simulink model "PTMotorCU"  (Simulink 8.7)
settings: Solver=ode45  StartTime=0.0  StopTime=inf  RelTol=1e-3
PreLoadFcn:
  | xData = [0 13.5 21 35 50 100];
  | yData = [150 150 95 57 39 20];
InitFcn:
  | xData = [0 0.128];
  | yData = [150 150];
libraries: simulink x6
(part 2 of 2)

== system PTMotorCU/CarMaker/IPG Vehicle/CarAndTrailer/Forces/Tires ==
  note: The TireXX_Out signals will only be used if FileIdent is "CarMaker-Tire-CM4SL" in the tire parameter file!
      | An example parameter file can be found in Data/Tire/DT_CM4SL_UserTire.
  Sync_In : Inport
  TireFL_In : Inport  Port=2
  TireFR_In : Inport  Port=3
  TireRL_In : Inport  Port=4
  TireRR_In : Inport  Port=5
  Bus Creator{1..4} (4 alike) : BusCreator  Inputs=11
  Demux{1..3,8} (4 alike) : Demux  Outputs=7
  TireFL : Subsystem
  TireFR : Subsystem
  TireRL : Subsystem
  TireRR : Subsystem
  TireFL_Out : Outport
  TireFR_Out : Outport  Port=2
  TireRL_Out : Outport  Port=3
  TireRR_Out : Outport  Port=4
  wires:
  Sync_In/1 -> TireRR/1(Sync_In), TireRL/1(Sync_In), TireFR/1(Sync_In), TireFL/1(Sync_In)
  Bus Creator4/1 -> TireRR_Out/1
  Bus Creator2/1 -> TireRL_Out/1
  Bus Creator1/1 -> TireFR_Out/1
  Demux3/5 -> TireRR/6(Rim_turnv)  "Tire_In Rim_turnv"
  Demux3/4 -> TireRR/5(Rim_rotv)  "Tire_In Rim_rotv"
  Demux3/1 -> TireRR/2(Load)  "Tire_In Load"
  Demux3/7 -> TireRR/8(muRoad)  "Tire_In mu"
  Demux3/6 -> TireRR/7(InclinAngle)  "Tire_In Camber"
  Demux3/2 -> TireRR/3(vxtrans)  "Tire_In vxtrans"
  Demux3/3 -> TireRR/4(vytrans)  "Tire_In vytrans"
  TireRR/11(AlignTrq) -> Bus Creator4/11  "Tire_Out AlignTrq"
  TireRR/10(RollResist) -> Bus Creator4/10  "Tire_Out RollResist"
  TireRR/9(OverturnTrq) -> Bus Creator4/9  "Tire_Out OverturnTrq"
  TireRR/8(LoadFrc) -> Bus Creator4/8  "Tire_Out LoadFrc"
  TireRR/7(SideFrc) -> Bus Creator4/7  "Tire_Out SideFrc"
  TireRR/6(LongFrc) -> Bus Creator4/6  "Tire_Out LongFrc"
  TireRR/5(vBelt) -> Bus Creator4/5  "Tire_Out vBelt"
  TireRR/4(rBelt_eff) -> Bus Creator4/4  "Tire_Out rBelt_eff"
  TireRR/3(TurnSlp) -> Bus Creator4/3  "Tire_Out TurnSlp"
  TireRR/1(Slp) -> Bus Creator4/1  "Tire_Out Slp"
  TireRR/2(Alpha) -> Bus Creator4/2  "Tire_Out Alpha"
  Demux2/5 -> TireRL/6(Rim_turnv)  "Tire_In Rim_turnv"
  Demux2/4 -> TireRL/5(Rim_rotv)  "Tire_In Rim_rotv"
  Demux2/1 -> TireRL/2(Load)  "Tire_In Load"
  Demux2/7 -> TireRL/8(muRoad)  "Tire_In mu"
  Demux2/6 -> TireRL/7(InclinAngle)  "Tire_In Camber"
  Demux2/2 -> TireRL/3(vxtrans)  "Tire_In vxtrans"
  Demux2/3 -> TireRL/4(vytrans)  "Tire_In vytrans"
  TireRL/11(AlignTrq) -> Bus Creator2/11  "Tire_Out AlignTrq"
  TireRL/10(RollResist) -> Bus Creator2/10  "Tire_Out RollResist"
  TireRL/9(OverturnTrq) -> Bus Creator2/9  "Tire_Out OverturnTrq"
  TireRL/8(LoadFrc) -> Bus Creator2/8  "Tire_Out LoadFrc"
  TireRL/7(SideFrc) -> Bus Creator2/7  "Tire_Out SideFrc"
  TireRL/6(LongFrc) -> Bus Creator2/6  "Tire_Out LongFrc"
  TireRL/5(vBelt) -> Bus Creator2/5  "Tire_Out vBelt"
  TireRL/4(rBelt_eff) -> Bus Creator2/4  "Tire_Out rBelt_eff"
  TireRL/3(TurnSlp) -> Bus Creator2/3  "Tire_Out TurnSlp"
  TireRL/1(Slp) -> Bus Creator2/1  "Tire_Out Slp"
  TireRL/2(Alpha) -> Bus Creator2/2  "Tire_Out Alpha"
  Demux1/5 -> TireFR/6(Rim_turnv)  "Tire_In Rim_turnv"
  Demux1/4 -> TireFR/5(Rim_rotv)  "Tire_In Rim_rotv"
  Demux1/1 -> TireFR/2(Load)  "Tire_In Load"
  Demux1/7 -> TireFR/8(muRoad)  "Tire_In mu"
  Demux1/6 -> TireFR/7(InclinAngle)  "Tire_In Camber"
  Demux1/2 -> TireFR/3(vxtrans)  "Tire_In vxtrans"
  Demux1/3 -> TireFR/4(vytrans)  "Tire_In vytrans"
  TireFR/11(AlignTrq) -> Bus Creator1/11  "Tire_Out AlignTrq"
  TireFR/10(RollResist) -> Bus Creator1/10  "Tire_Out RollResist"
  TireFR/9(OverturnTrq) -> Bus Creator1/9  "Tire_Out OverturnTrq"
  TireFR/8(LoadFrc) -> Bus Creator1/8  "Tire_Out LoadFrc"
  TireFR/7(SideFrc) -> Bus Creator1/7  "Tire_Out SideFrc"
  TireFR/6(LongFrc) -> Bus Creator1/6  "Tire_Out LongFrc"
  TireFR/5(vBelt) -> Bus Creator1/5  "Tire_Out vBelt"
  TireFR/4(rBelt_eff) -> Bus Creator1/4  "Tire_Out rBelt_eff"
  TireFR/3(TurnSlp) -> Bus Creator1/3  "Tire_Out TurnSlp"
  TireFR/1(Slp) -> Bus Creator1/1  "Tire_Out Slp"
  TireFR/2(Alpha) -> Bus Creator1/2  "Tire_Out Alpha"
  Demux8/5 -> TireFL/6(Rim_turnv)  "Tire_In Rim_turnv"
  Demux8/4 -> TireFL/5(Rim_rotv)  "Tire_In Rim_rotv"
  TireFL_In/1 -> Demux8/1
  Demux8/1 -> TireFL/2(Load)  "Tire_In Load"
  Demux8/7 -> TireFL/8(muRoad)  "Tire_In mu"
  Demux8/6 -> TireFL/7(InclinAngle)  "Tire_In Camber"
  Demux8/2 -> TireFL/3(vxtrans)  "Tire_In vxtrans"
  Demux8/3 -> TireFL/4(vytrans)  "Tire_In vytrans"
  TireFL/11(AlignTrq) -> Bus Creator3/11  "Tire_Out AlignTrq"
  TireFL/10(RollResist) -> Bus Creator3/10  "Tire_Out RollResist"
  TireFL/9(OverturnTrq) -> Bus Creator3/9  "Tire_Out OverturnTrq"
  TireFL/8(LoadFrc) -> Bus Creator3/8  "Tire_Out LoadFrc"
  TireFL/7(SideFrc) -> Bus Creator3/7  "Tire_Out SideFrc"
  TireFL/6(LongFrc) -> Bus Creator3/6  "Tire_Out LongFrc"
  TireFL/5(vBelt) -> Bus Creator3/5  "Tire_Out vBelt"
  TireFL/4(rBelt_eff) -> Bus Creator3/4  "Tire_Out rBelt_eff"
  TireFL/3(TurnSlp) -> Bus Creator3/3  "Tire_Out TurnSlp"
  TireFL/1(Slp) -> Bus Creator3/1  "Tire_Out Slp"
  TireFL/2(Alpha) -> Bus Creator3/2  "Tire_Out Alpha"
  Bus Creator3/1 -> TireFL_Out/1
  TireFR_In/1 -> Demux1/1
  TireRL_In/1 -> Demux2/1
  TireRR_In/1 -> Demux3/1

== system PTMotorCU/CarMaker/IPG Vehicle/CarAndTrailer/Forces/Vehicle Forces ==
  Sync_In : Inport
  Bus Creator1 : BusCreator  Inputs=12
  Bus Creator8 : BusCreator  Inputs=16
  BusCreator1 : BusCreator  Inputs=4
  BusCreator2 : BusCreator  Inputs=9
  Demux : Demux  Outputs=16
  Demux1 : Demux  Outputs=12
  Demux2 : Demux  Outputs=13
  Forces : S-Function  FunctionName=CM_Sfun  Parameters='Forces'  SFunctionDeploymentMode=off  EnableBusSupport=off
  Terminator : Terminator
  Sync_Out : Outport
  Car.Virtual : Outport  Port=2
  Car.Aero : Outport  Port=3
  Car.Load : Outport  Port=4
  wires:
  BusCreator1/1 -> Terminator/1  "Aero IF (in)"
  Demux2/13 -> BusCreator2/9  "car Aero Trq_1 z"
  Demux2/12 -> BusCreator2/8  "car Aero Trq_1 y"
  Demux2/11 -> BusCreator2/7  "car Aero Trq_1 x"
  Demux2/10 -> BusCreator2/6  "car Aero Frc_1 z"
  Demux2/9 -> BusCreator2/5  "car Aero Frc_1 y"
  Demux2/8 -> BusCreator2/4  "car Aero Frc_1 x"
  Demux2/7 -> BusCreator2/3  "car Aero PoA_1 z"
  Demux2/6 -> BusCreator2/2  "car Aero PoA_1 y"
  Demux2/5 -> BusCreator2/1  "car Aero PoA_1 x"
  Demux2/4 -> BusCreator1/4  "car Aero tau_1"
  Demux2/3 -> BusCreator1/3  "car Aero ApproachVel_1 z"
  Demux2/2 -> BusCreator1/2  "car Aero ApproachVel_1 y"
  Demux2/1 -> BusCreator1/1  "car Aero ApproachVel_1 x"
  Demux/16 -> Bus Creator8/16  "Car Load_3 tz"
  Demux/15 -> Bus Creator8/15  "Car Load_3 ty"
  Demux/14 -> Bus Creator8/14  "Car Load_3 tx"
  Demux/13 -> Bus Creator8/13  "Car Load_3 mass"
  Demux1/12 -> Bus Creator1/12  "Car Virtual Trq_0 z"
  Demux1/11 -> Bus Creator1/11  "Car Virtual Trq_0 y"
  Demux1/10 -> Bus Creator1/10  "Car Virtual Trq_0 x"
  Demux1/9 -> Bus Creator1/9  "Car Virtual Trq_1 z"
  Demux1/8 -> Bus Creator1/8  "Car Virtual Trq_1 y"
  Demux1/7 -> Bus Creator1/7  "Car Virtual Trq_1 x"
  Demux1/6 -> Bus Creator1/6  "Car Virtual Frc_0 z"
  Demux1/5 -> Bus Creator1/5  "Car Virtual Frc_0 y"
  Demux1/4 -> Bus Creator1/4  "Car Virtual Frc_0 x"
  Sync_In/1 -> Forces/1
  Forces/1 -> Sync_Out/1
  BusCreator2/1 -> Car.Aero/1
  Demux1/1 -> Bus Creator1/1  "Car Virtual Frc_1 x"
  Demux1/2 -> Bus Creator1/2  "Car Virtual Frc_1 y"
  Demux1/3 -> Bus Creator1/3  "Car Virtual Frc_1 z"
  Forces/3 -> Demux2/1
  Forces/2 -> Demux1/1
  Bus Creator1/1 -> Car.Virtual/1
  Bus Creator8/1 -> Car.Load/1
  Demux/1 -> Bus Creator8/1  "Car Load_0 mass"
  Demux/2 -> Bus Creator8/2  "Car Load_0 tx"
  Demux/3 -> Bus Creator8/3  "Car Load_0 ty"
  Demux/4 -> Bus Creator8/4  "Car Load_0 tz"
  Demux/5 -> Bus Creator8/5  "Car Load_1 mass"
  Demux/6 -> Bus Creator8/6  "Car Load_1 tx"
  Demux/7 -> Bus Creator8/7  "Car Load_1 ty"
  Demux/8 -> Bus Creator8/8  "Car Load_1 tz"
  Demux/9 -> Bus Creator8/9  "Car Load_2 mass"
  Demux/10 -> Bus Creator8/10  "Car Load_2 tx"
  Demux/11 -> Bus Creator8/11  "Car Load_2 ty"
  Demux/12 -> Bus Creator8/12  "Car Load_2 tz"
  Forces/4 -> Demux/1

== system PTMotorCU/CarMaker/IPG Vehicle/CarAndTrailer/Trailer/CreateBus Car.Hitch.FrcTrq ==
  In1 : Inport
  Bus Creator7 : BusCreator  Inputs=6
  Demux7 : Demux  Outputs=6
  Out1 : Outport
  wires:
  In1/1 -> Demux7/1
  Bus Creator7/1 -> Out1/1
  Demux7/6 -> Bus Creator7/6  "Car Hitch Trq2Car z"
  Demux7/5 -> Bus Creator7/5  "Car Hitch Trq2Car y"
  Demux7/4 -> Bus Creator7/4  "Car Hitch Trq2Car x"
  Demux7/3 -> Bus Creator7/3  "Car Hitch Frc2Car z"
  Demux7/2 -> Bus Creator7/2  "Car Hitch Frc2Car y"
  Demux7/1 -> Bus Creator7/1  "Car Hitch Frc2Car x"

== system PTMotorCU/CarMaker/IPG Vehicle/CarAndTrailer/Trailer/CreateBus Vhcl.Motion ==
  In1 : Inport
  BusCreator : BusCreator  Inputs=15
  Demux : Demux  Outputs=15
  Out1 : Outport
  wires:
  Demux/15 -> BusCreator/15  "Vhcl YawAcc"
  Demux/14 -> BusCreator/14  "Vhcl YawVel"
  Demux/13 -> BusCreator/13  "Vhcl Yaw"
  Demux/12 -> BusCreator/12  "Vhcl PitchAcc"
  Demux/11 -> BusCreator/11  "Vhcl PitchVel"
  Demux/10 -> BusCreator/10  "Vhcl Pitch"
  Demux/9 -> BusCreator/9  "Vhcl RollAcc"
  Demux/8 -> BusCreator/8  "Vhcl RollVel"
  Demux/7 -> BusCreator/7  "Vhcl Roll"
  Demux/6 -> BusCreator/6  "Vhcl Hitch_Pos z"
  Demux/5 -> BusCreator/5  "Vhcl Hitch_Pos y"
  Demux/4 -> BusCreator/4  "Vhcl Hitch_Pos x"
  Demux/3 -> BusCreator/3  "Vhcl sRoad"
  Demux/2 -> BusCreator/2  "Vhcl Distance"
  Demux/1 -> BusCreator/1  "Vhcl v"
  In1/1 -> Demux/1
  BusCreator/1 -> Out1/1

== system PTMotorCU/CarMaker/IPG Vehicle/CarAndTrailer/Trailer/CreateBus Vhcl.PoI ==
  In1 : Inport
  Bus Creator3 : BusCreator  Inputs=18
  Demux3 : Demux  Outputs=18
  Out1 : Outport
  wires:
  Demux3/18 -> Bus Creator3/18  "Vhcl PoI_GCS Elev"
  Demux3/17 -> Bus Creator3/17  "Vhcl PoI_GCS Lat"
  Demux3/16 -> Bus Creator3/16  "Vhcl PoI_GCS Long"
  Demux3/15 -> Bus Creator3/15  "Vhcl PoI_Acc_1 z"
  Demux3/14 -> Bus Creator3/14  "Vhcl PoI_Acc_1 y"
  Demux3/13 -> Bus Creator3/13  "Vhcl PoI_Acc_1 x"
  Demux3/12 -> Bus Creator3/12  "Vhcl PoI_Vel_1 z"
  Demux3/11 -> Bus Creator3/11  "Vhcl PoI_Vel_1 y"
  Demux3/10 -> Bus Creator3/10  "Vhcl PoI_Vel_1 x"
  Demux3/9 -> Bus Creator3/9  "Vhcl PoI_Acc z"
  Demux3/8 -> Bus Creator3/8  "Vhcl PoI_Acc y"
  Demux3/7 -> Bus Creator3/7  "Vhcl PoI_Acc x"
  Demux3/6 -> Bus Creator3/6  "Vhcl PoI_Vel z"
  Demux3/5 -> Bus Creator3/5  "Vhcl PoI_Vel y"
  Demux3/4 -> Bus Creator3/4  "Vhcl PoI_Vel x"
  Demux3/3 -> Bus Creator3/3  "Vhcl PoI_Pos z"
  Demux3/2 -> Bus Creator3/2  "Vhcl PoI_Pos y"
  In1/1 -> Demux3/1
  Bus Creator3/1 -> Out1/1
  Demux3/1 -> Bus Creator3/1  "Vhcl PoI_Pos x"

== system PTMotorCU/CarMaker/IPG Vehicle/CarAndTrailer/Trailer/CreateBus Vhcl.Steering ==
  In1 : Inport
  Bus Creator3 : BusCreator  Inputs=4
  Demux : Demux
  Out1 : Outport
  wires:
  Bus Creator3/1 -> Out1/1
  Demux/1 -> Bus Creator3/1  "Vhcl Steering Ang"
  Demux/3 -> Bus Creator3/3  "Vhcl Steering AngAcc"
  Demux/2 -> Bus Creator3/2  "Vhcl Steering AngVel"
  Demux/4 -> Bus Creator3/4  "Vhcl Steering Trq"
  In1/1 -> Demux/1

== system PTMotorCU/CarMaker/IPG Vehicle/CarAndTrailer/Trailer/CreateBus Vhcl.Wheel.FL ==
  In1 : Inport
  Bus Creator3 : BusCreator  Inputs=14
  Demux3 : Demux  Outputs=14
  Out1 : Outport
  wires:
  Demux3/14 -> Bus Creator3/14  "Vhcl Wheel FL Trq_WhlBearing"
  Demux3/13 -> Bus Creator3/13  "Vhcl Wheel FL Trq_T2W"
  Demux3/12 -> Bus Creator3/12  "Vhcl Wheel FL SideSlip"
  Demux3/11 -> Bus Creator3/11  "Vhcl Wheel FL LongSlip"
  Demux3/10 -> Bus Creator3/10  "Vhcl Wheel FL vBelt"
  Demux3/9 -> Bus Creator3/9  "Vhcl Wheel FL Fz"
  Demux3/8 -> Bus Creator3/8  "Vhcl Wheel FL Fy"
  Demux3/7 -> Bus Creator3/7  "Vhcl Wheel FL Fx"
  Demux3/6 -> Bus Creator3/6  "Vhcl Wheel FL r_zxy z"
  Demux3/5 -> Bus Creator3/5  "Vhcl Wheel FL r_zxy y"
  Demux3/4 -> Bus Creator3/4  "Vhcl Wheel FL r_zxy x"
  Demux3/3 -> Bus Creator3/3  "Vhcl Wheel FL t z"
  Demux3/2 -> Bus Creator3/2  "Vhcl Wheel FL t y"
  In1/1 -> Demux3/1
  Bus Creator3/1 -> Out1/1
  Demux3/1 -> Bus Creator3/1  "Vhcl Wheel FL t x"

== system PTMotorCU/CarMaker/IPG Vehicle/CarAndTrailer/Trailer/CreateBus Vhcl.Wheel.FR ==
  In1 : Inport
  Bus Creator3 : BusCreator  Inputs=14
  Demux3 : Demux  Outputs=14
  Out1 : Outport
  wires:
  Demux3/14 -> Bus Creator3/14  "Vhcl Wheel FR Trq_WhlBearing"
  Demux3/13 -> Bus Creator3/13  "Vhcl Wheel FR Trq_T2W"
  Demux3/12 -> Bus Creator3/12  "Vhcl Wheel FR SideSlip"
  Demux3/11 -> Bus Creator3/11  "Vhcl Wheel FR LongSlip"
  Demux3/10 -> Bus Creator3/10  "Vhcl Wheel FR vBelt"
  Demux3/9 -> Bus Creator3/9  "Vhcl Wheel FR Fz"
  Demux3/8 -> Bus Creator3/8  "Vhcl Wheel FR Fy"
  Demux3/7 -> Bus Creator3/7  "Vhcl Wheel FR Fx"
  Demux3/6 -> Bus Creator3/6  "Vhcl Wheel FR r_zxy z"
  Demux3/5 -> Bus Creator3/5  "Vhcl Wheel FR r_zxy y"
  Demux3/4 -> Bus Creator3/4  "Vhcl Wheel FR r_zxy x"
  Demux3/3 -> Bus Creator3/3  "Vhcl Wheel FR t z"
  Demux3/2 -> Bus Creator3/2  "Vhcl Wheel FR t y"
  In1/1 -> Demux3/1
  Bus Creator3/1 -> Out1/1
  Demux3/1 -> Bus Creator3/1  "Vhcl Wheel FR t x"

== system PTMotorCU/CarMaker/IPG Vehicle/CarAndTrailer/Trailer/CreateBus Vhcl.Wheel.RL ==
  In1 : Inport
  Bus Creator3 : BusCreator  Inputs=14
  Demux3 : Demux  Outputs=14
  Out1 : Outport
  wires:
  Demux3/14 -> Bus Creator3/14  "Vhcl Wheel RL Trq_WhlBearing"
  Demux3/13 -> Bus Creator3/13  "Vhcl Wheel RL Trq_T2W"
  Demux3/12 -> Bus Creator3/12  "Vhcl Wheel RL SideSlip"
  Demux3/11 -> Bus Creator3/11  "Vhcl Wheel RL LongSlip"
  Demux3/10 -> Bus Creator3/10  "Vhcl Wheel RL vBelt"
  Demux3/9 -> Bus Creator3/9  "Vhcl Wheel RL Fz"
  Demux3/8 -> Bus Creator3/8  "Vhcl Wheel RL Fy"
  Demux3/7 -> Bus Creator3/7  "Vhcl Wheel RL Fx"
  Demux3/6 -> Bus Creator3/6  "Vhcl Wheel RL r_zxy z"
  Demux3/5 -> Bus Creator3/5  "Vhcl Wheel RL r_zxy y"
  Demux3/4 -> Bus Creator3/4  "Vhcl Wheel RL r_zxy x"
  Demux3/3 -> Bus Creator3/3  "Vhcl Wheel RL t z"
  Demux3/2 -> Bus Creator3/2  "Vhcl Wheel RL t y"
  In1/1 -> Demux3/1
  Bus Creator3/1 -> Out1/1
  Demux3/1 -> Bus Creator3/1  "Vhcl Wheel RL t x"

== system PTMotorCU/CarMaker/IPG Vehicle/CarAndTrailer/Trailer/CreateBus Vhcl.Wheel.RR ==
  In1 : Inport
  Bus Creator3 : BusCreator  Inputs=14
  Demux3 : Demux  Outputs=14
  Out1 : Outport
  wires:
  Demux3/14 -> Bus Creator3/14  "Vhcl Wheel RR Trq_WhlBearing"
  Demux3/13 -> Bus Creator3/13  "Vhcl Wheel RR Trq_T2W"
  Demux3/12 -> Bus Creator3/12  "Vhcl Wheel RR SideSlip"
  Demux3/11 -> Bus Creator3/11  "Vhcl Wheel RR LongSlip"
  Demux3/10 -> Bus Creator3/10  "Vhcl Wheel RR vBelt"
  Demux3/9 -> Bus Creator3/9  "Vhcl Wheel RR Fz"
  Demux3/8 -> Bus Creator3/8  "Vhcl Wheel RR Fy"
  Demux3/7 -> Bus Creator3/7  "Vhcl Wheel RR Fx"
  Demux3/6 -> Bus Creator3/6  "Vhcl Wheel RR r_zxy z"
  Demux3/5 -> Bus Creator3/5  "Vhcl Wheel RR r_zxy y"
  Demux3/4 -> Bus Creator3/4  "Vhcl Wheel RR r_zxy x"
  Demux3/3 -> Bus Creator3/3  "Vhcl Wheel RR t z"
  Demux3/2 -> Bus Creator3/2  "Vhcl Wheel RR t y"
  In1/1 -> Demux3/1
  Bus Creator3/1 -> Out1/1
  Demux3/1 -> Bus Creator3/1  "Vhcl Wheel RR t x"

== system PTMotorCU/CarMaker/IPG Vehicle/PowerTrain/MCU Example/CreateBus MCU ISGOut ==
  In : Inport
  BusCreator : BusCreator  Inputs=3
  Demux : Demux  Outputs=3
  Out : Outport
  wires:
  Demux/3 -> BusCreator/3  "MCU ISGOut TrqGen_max"
  Demux/2 -> BusCreator/2  "MCU ISGOut TrqMot_max"
  Demux/1 -> BusCreator/1  "MCU ISGOut Load"
  BusCreator/1 -> Out/1
  In/1 -> Demux/1

== system PTMotorCU/CarMaker/IPG Vehicle/PowerTrain/MCU Example/CreateBus MCU MotorOut0 ==
  In : Inport
  BusCreator : BusCreator  Inputs=3
  Demux : Demux  Outputs=3
  Out : Outport
  wires:
  Demux/3 -> BusCreator/3  "MCU MotorOut0 TrqGen_max"
  Demux/2 -> BusCreator/2  "MCU MotorOut0 TrqMot_max"
  Demux/1 -> BusCreator/1  "MCU MotorOut0 Load"
  BusCreator/1 -> Out/1
  In/1 -> Demux/1

== system PTMotorCU/CarMaker/IPG Vehicle/PowerTrain/MCU Example/CreateBus MCU MotorOut1 ==
  In : Inport
  BusCreator : BusCreator  Inputs=3
  Demux : Demux  Outputs=3
  Out : Outport
  wires:
  Demux/3 -> BusCreator/3  "MCU MotorOut1 TrqGen_max"
  Demux/2 -> BusCreator/2  "MCU MotorOut1 TrqMot_max"
  Demux/1 -> BusCreator/1  "MCU MotorOut1 Load"
  BusCreator/1 -> Out/1
  In/1 -> Demux/1

== system PTMotorCU/CarMaker/IPG Vehicle/PowerTrain/MCU Example/CreateBus MCU MotorOut2 ==
  In : Inport
  BusCreator : BusCreator  Inputs=3
  Demux : Demux  Outputs=3
  Out : Outport
  wires:
  Demux/3 -> BusCreator/3  "MCU MotorOut2 TrqGen_max"
  Demux/2 -> BusCreator/2  "MCU MotorOut2 TrqMot_max"
  Demux/1 -> BusCreator/1  "MCU MotorOut2 Load"
  BusCreator/1 -> Out/1
  In/1 -> Demux/1

== system PTMotorCU/CarMaker/IPG Vehicle/PowerTrain/MCU Example/CreateBus MCU MotorOut3 ==
  In : Inport
  BusCreator : BusCreator  Inputs=3
  Demux : Demux  Outputs=3
  Out : Outport
  wires:
  Demux/3 -> BusCreator/3  "MCU MotorOut3 TrqGen_max"
  Demux/2 -> BusCreator/2  "MCU MotorOut3 TrqMot_max"
  Demux/1 -> BusCreator/1  "MCU MotorOut3 Load"
  BusCreator/1 -> Out/1
  In/1 -> Demux/1

== system PTMotorCU/CarMaker/IPG Vehicle/PowerTrain/MCU Example/CreateBus MCU Status ==
  In : Inport
  BusCreator : BusCreator  Inputs=1
  Demux : Demux  Outputs=1
  Out : Outport
  wires:
  Demux/1 -> BusCreator/1  "MCU_Out Status"
  BusCreator/1 -> Out/1
  In/1 -> Demux/1

== system PTMotorCU/CarMaker/IPG Vehicle/PowerTrain/MCU Example/MyMotorCU ==
  Ignition : Inport
  rotv : Inport  Port=2
  Trq_trg : Inport  Port=3
  Load : Inport  Port=4
  rotv_trg : Inport  Port=5
  CfgIF : Inport  Port=6
  Bus Creator : BusCreator  Inputs=3
  Bus Selector : BusSelector  OutputSignals=MCU_Cfg ISG Ratio,TrqMot_max ,TrqGen_max,MCU_Cfg ISG rotv_Mot_max,MCU_Cfg ISG rotv_Gen_max
  Bus Selector1 : BusSelector  OutputSignals=Load,TrqMot_max,TrqGen_max
  Enabled Subsystem : Subsystem  TreatAsAtomicUnit=on
  Logical Operator : Logic  Operator=NOT  AllPortsSameDT=off  OutDataTypeStr=boolean
  Merge : Merge
  ReturnZero : Subsystem  TreatAsAtomicUnit=on
  Load out : Outport
  TrqMot_max : Outport  Port=2
  TrqGen_max : Outport  Port=3
  wires:
  Bus Selector1/1 -> Load out/1  "<Load>"
  Bus Selector1/2 -> TrqMot_max/1  "<TrqMot_max>"
  Bus Selector1/3 -> TrqGen_max/1  "<TrqGen_max>"
  Merge/1 -> Bus Selector1/1
  Bus Creator/1 -> Merge/2
  ReturnZero/1(ReturnZero) -> Merge/1
  Enabled Subsystem/3(TrqGen_max) -> Bus Creator/3  "TrqGen_max"
  Enabled Subsystem/2(TrqMot_max) -> Bus Creator/2  "TrqMot_max"
  Enabled Subsystem/1(Load out) -> Bus Creator/1  "Load"
  rotv_trg/1 -> Enabled Subsystem/4(rotv_trg)
  Load/1 -> Enabled Subsystem/3(Load)
  Trq_trg/1 -> Enabled Subsystem/2(Trq_trg)
  Bus Selector/5 -> Enabled Subsystem/9(rotv_Gen_max)  "<MCU_Cfg ISG rotv_Gen_max>"
  Bus Selector/4 -> Enabled Subsystem/8(rotv_Mot_max)  "<MCU_Cfg ISG rotv_Mot_max>"
  Bus Selector/3 -> Enabled Subsystem/7(TrqGen_max table)  "<TrqGen_max>"
  Bus Selector/2 -> Enabled Subsystem/6(TrqMot_max table)  "<TrqMot_max >"
  Bus Selector/1 -> Enabled Subsystem/5(Ratio)  "<MCU_Cfg ISG Ratio>"
  CfgIF/1 -> Bus Selector/1
  rotv/1 -> Enabled Subsystem/1(rotv)
  Logical Operator/1 -> ReturnZero/Enable
  Ignition/1 -> Logical Operator/1, Enabled Subsystem/Enable

== system PTMotorCU/CarMaker/IPG Vehicle/PowerTrain/MCU Example/PTMotorCU_In ==
  Sync_In : Inport
  CreateBus MCU ISGIn : Subsystem
  CreateBus MCU ISGOut : Subsystem
  CreateBus MCU Ignition : Subsystem
  CreateBus MCU MotorIn0 : Subsystem
  CreateBus MCU MotorIn1 : Subsystem
  CreateBus MCU MotorIn2 : Subsystem
  CreateBus MCU MotorIn3 : Subsystem
  CreateBus MCU MotorOut0 : Subsystem
  CreateBus MCU MotorOut1 : Subsystem
  CreateBus MCU MotorOut2 : Subsystem
  CreateBus MCU MotorOut3 : Subsystem
  CreateBus MCU_Cfg ISG : Subsystem
  CreateBus MCU_Cfg Misc : Subsystem
  CreateBus MCU_Cfg Motor0 : Subsystem
  CreateBus MCU_Cfg Motor1 : Subsystem
  CreateBus MCU_Cfg Motor2 : Subsystem
  CreateBus MCU_Cfg Motor3 : Subsystem
  CreateBus PTMotorCU_In : BusCreator  Inputs=17
  S-Function : S-Function  FunctionName=cm_ptmotorcu_in  SFunctionDeploymentMode=off  EnableBusSupport=off
  PTMotorCU_In : Outport
  wires:
  CreateBus MCU MotorOut3/1(Out) -> CreateBus PTMotorCU_In/17  "MCU MotorOut3"
  S-Function/17 -> CreateBus MCU MotorOut3/1(In)
  CreateBus MCU MotorOut2/1(Out) -> CreateBus PTMotorCU_In/16  "MCU MotorOut2"
  S-Function/16 -> CreateBus MCU MotorOut2/1(In)
  CreateBus MCU MotorOut1/1(Out) -> CreateBus PTMotorCU_In/15  "MCU MotorOut1"
  S-Function/15 -> CreateBus MCU MotorOut1/1(In)
  CreateBus MCU MotorOut0/1(Out) -> CreateBus PTMotorCU_In/14  "MCU MotorOut0"
  S-Function/14 -> CreateBus MCU MotorOut0/1(In)
  CreateBus MCU MotorIn3/1(Out) -> CreateBus PTMotorCU_In/13  "MCU MotorIn3"
  S-Function/13 -> CreateBus MCU MotorIn3/1(In)
  CreateBus MCU MotorIn2/1(Out) -> CreateBus PTMotorCU_In/12  "MCU MotorIn2"
  S-Function/12 -> CreateBus MCU MotorIn2/1(In)
  CreateBus MCU MotorIn1/1(Out) -> CreateBus PTMotorCU_In/11  "MCU MotorIn1"
  S-Function/11 -> CreateBus MCU MotorIn1/1(In)
  CreateBus MCU MotorIn0/1(Out) -> CreateBus PTMotorCU_In/10  "MCU MotorIn0"
  S-Function/10 -> CreateBus MCU MotorIn0/1(In)
  CreateBus MCU ISGOut/1(Out) -> CreateBus PTMotorCU_In/9  "MCU ISGOut"
  S-Function/9 -> CreateBus MCU ISGOut/1(In)
  CreateBus MCU ISGIn/1(Out) -> CreateBus PTMotorCU_In/8  "MCU ISGIn"
  S-Function/8 -> CreateBus MCU ISGIn/1(In)
  CreateBus MCU Ignition/1(Out) -> CreateBus PTMotorCU_In/7  "MCU Ignition"
  S-Function/7 -> CreateBus MCU Ignition/1(In)
  CreateBus MCU_Cfg Motor3/1(Out) -> CreateBus PTMotorCU_In/6  "MCU_Cfg Motor3"
  S-Function/6 -> CreateBus MCU_Cfg Motor3/1(In)
  CreateBus MCU_Cfg Motor2/1(Out) -> CreateBus PTMotorCU_In/5  "MCU_Cfg Motor2"
  S-Function/5 -> CreateBus MCU_Cfg Motor2/1(In)
  CreateBus MCU_Cfg Motor1/1(Out) -> CreateBus PTMotorCU_In/4  "MCU_Cfg Motor1"
  S-Function/4 -> CreateBus MCU_Cfg Motor1/1(In)
  CreateBus MCU_Cfg Motor0/1(Out) -> CreateBus PTMotorCU_In/3  "MCU_Cfg Motor0"
  S-Function/3 -> CreateBus MCU_Cfg Motor0/1(In)
  CreateBus MCU_Cfg ISG/1(Out) -> CreateBus PTMotorCU_In/2  "MCU_Cfg ISG"
  S-Function/2 -> CreateBus MCU_Cfg ISG/1(In)
  CreateBus MCU_Cfg Misc/1(Out) -> CreateBus PTMotorCU_In/1  "MCU_Cfg Misc"
  S-Function/1 -> CreateBus MCU_Cfg Misc/1(In)
  CreateBus PTMotorCU_In/1 -> PTMotorCU_In/1
  Sync_In/1 -> S-Function/1

== system PTMotorCU/CarMaker/IPG Vehicle/PowerTrain/MCU Example/PTMotorCU_Out ==
  MCU Status : Inport
  MCU ISGOut : Inport  Port=2
  MCU MotorOut0 : Inport  Port=3
  MCU MotorOut1 : Inport  Port=4
  MCU MotorOut2 : Inport  Port=5
  MCU MotorOut3 : Inport  Port=6
  S-Function : S-Function  FunctionName=cm_ptmotorcu_out  SFunctionDeploymentMode=off  EnableBusSupport=off
  wires:
  MCU MotorOut3/1 -> S-Function/6
  MCU MotorOut2/1 -> S-Function/5
  MCU MotorOut1/1 -> S-Function/4
  MCU MotorOut0/1 -> S-Function/3
  MCU ISGOut/1 -> S-Function/2
  MCU Status/1 -> S-Function/1

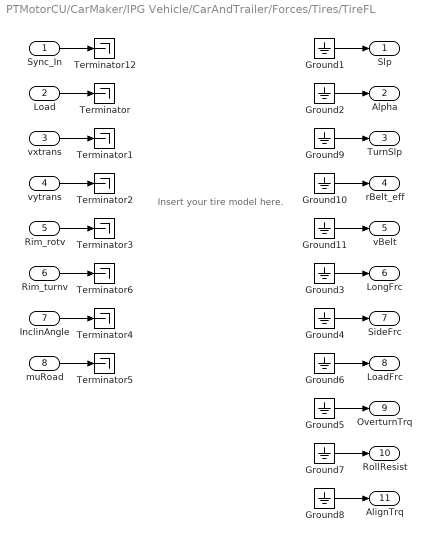
== system PTMotorCU/CarMaker/IPG Vehicle/CarAndTrailer/Forces/Tires/TireFL ==
  note: Insert your tire model here.
  Sync_In : Inport
  Load : Inport  Port=2
  vxtrans : Inport  Port=3
  vytrans : Inport  Port=4
  Rim_rotv : Inport  Port=5
  Rim_turnv : Inport  Port=6
  InclinAngle : Inport  Port=7
  muRoad : Inport  Port=8
  Ground{1..11} (11 alike) : Ground
  Terminator{,1..6,12} (8 alike) : Terminator
  Slp : Outport
  Alpha : Outport  Port=2
  TurnSlp : Outport  Port=3
  rBelt_eff : Outport  Port=4
  vBelt : Outport  Port=5
  LongFrc : Outport  Port=6
  SideFrc : Outport  Port=7
  LoadFrc : Outport  Port=8
  OverturnTrq : Outport  Port=9
  RollResist : Outport  Port=10
  AlignTrq : Outport  Port=11
  wires:
  Ground11/1 -> vBelt/1
  Ground10/1 -> rBelt_eff/1
  Ground9/1 -> TurnSlp/1
  Rim_turnv/1 -> Terminator6/1
  Sync_In/1 -> Terminator12/1
  Ground2/1 -> Alpha/1
  Ground3/1 -> LongFrc/1
  Ground4/1 -> SideFrc/1
  Ground5/1 -> OverturnTrq/1
  vxtrans/1 -> Terminator1/1
  vytrans/1 -> Terminator2/1
  Rim_rotv/1 -> Terminator3/1
  InclinAngle/1 -> Terminator4/1
  muRoad/1 -> Terminator5/1
  Load/1 -> Terminator/1
  Ground1/1 -> Slp/1
  Ground6/1 -> LoadFrc/1
  Ground7/1 -> RollResist/1
  Ground8/1 -> AlignTrq/1

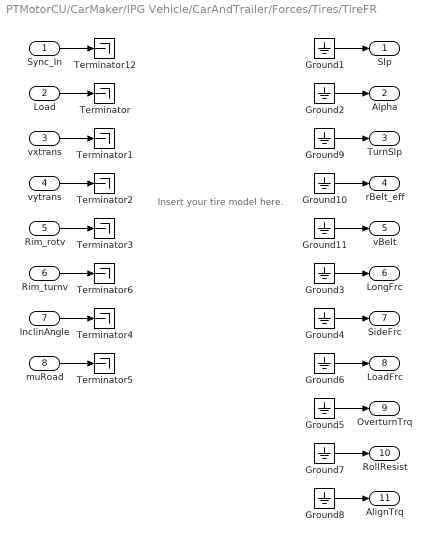
== system PTMotorCU/CarMaker/IPG Vehicle/CarAndTrailer/Forces/Tires/TireFR ==
  note: Insert your tire model here.
  Sync_In : Inport
  Load : Inport  Port=2
  vxtrans : Inport  Port=3
  vytrans : Inport  Port=4
  Rim_rotv : Inport  Port=5
  Rim_turnv : Inport  Port=6
  InclinAngle : Inport  Port=7
  muRoad : Inport  Port=8
  Ground{1..11} (11 alike) : Ground
  Terminator{,1..6,12} (8 alike) : Terminator
  Slp : Outport
  Alpha : Outport  Port=2
  TurnSlp : Outport  Port=3
  rBelt_eff : Outport  Port=4
  vBelt : Outport  Port=5
  LongFrc : Outport  Port=6
  SideFrc : Outport  Port=7
  LoadFrc : Outport  Port=8
  OverturnTrq : Outport  Port=9
  RollResist : Outport  Port=10
  AlignTrq : Outport  Port=11
  wires:
  Ground11/1 -> vBelt/1
  Ground10/1 -> rBelt_eff/1
  Ground9/1 -> TurnSlp/1
  Rim_turnv/1 -> Terminator6/1
  Sync_In/1 -> Terminator12/1
  Ground2/1 -> Alpha/1
  Ground3/1 -> LongFrc/1
  Ground4/1 -> SideFrc/1
  Ground5/1 -> OverturnTrq/1
  vxtrans/1 -> Terminator1/1
  vytrans/1 -> Terminator2/1
  Rim_rotv/1 -> Terminator3/1
  InclinAngle/1 -> Terminator4/1
  muRoad/1 -> Terminator5/1
  Load/1 -> Terminator/1
  Ground1/1 -> Slp/1
  Ground6/1 -> LoadFrc/1
  Ground7/1 -> RollResist/1
  Ground8/1 -> AlignTrq/1

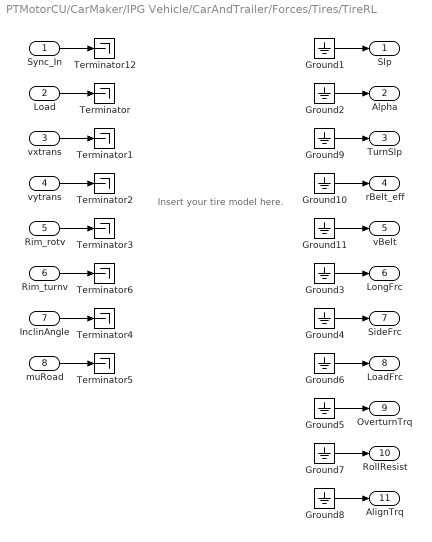
== system PTMotorCU/CarMaker/IPG Vehicle/CarAndTrailer/Forces/Tires/TireRL ==
  note: Insert your tire model here.
  Sync_In : Inport
  Load : Inport  Port=2
  vxtrans : Inport  Port=3
  vytrans : Inport  Port=4
  Rim_rotv : Inport  Port=5
  Rim_turnv : Inport  Port=6
  InclinAngle : Inport  Port=7
  muRoad : Inport  Port=8
  Ground{1..11} (11 alike) : Ground
  Terminator{,1..6,12} (8 alike) : Terminator
  Slp : Outport
  Alpha : Outport  Port=2
  TurnSlp : Outport  Port=3
  rBelt_eff : Outport  Port=4
  vBelt : Outport  Port=5
  LongFrc : Outport  Port=6
  SideFrc : Outport  Port=7
  LoadFrc : Outport  Port=8
  OverturnTrq : Outport  Port=9
  RollResist : Outport  Port=10
  AlignTrq : Outport  Port=11
  wires:
  Ground11/1 -> vBelt/1
  Ground10/1 -> rBelt_eff/1
  Ground9/1 -> TurnSlp/1
  Rim_turnv/1 -> Terminator6/1
  Sync_In/1 -> Terminator12/1
  Ground2/1 -> Alpha/1
  Ground3/1 -> LongFrc/1
  Ground4/1 -> SideFrc/1
  Ground5/1 -> OverturnTrq/1
  vxtrans/1 -> Terminator1/1
  vytrans/1 -> Terminator2/1
  Rim_rotv/1 -> Terminator3/1
  InclinAngle/1 -> Terminator4/1
  muRoad/1 -> Terminator5/1
  Load/1 -> Terminator/1
  Ground1/1 -> Slp/1
  Ground6/1 -> LoadFrc/1
  Ground7/1 -> RollResist/1
  Ground8/1 -> AlignTrq/1

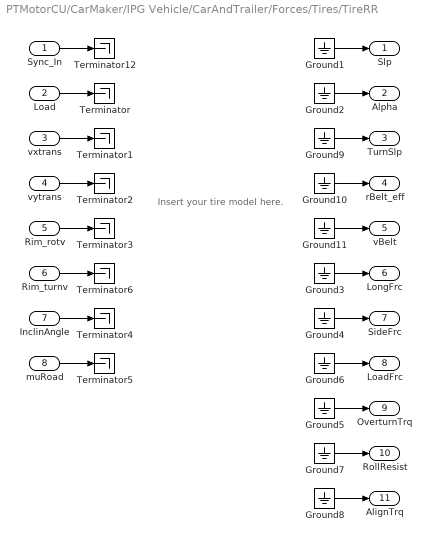
== system PTMotorCU/CarMaker/IPG Vehicle/CarAndTrailer/Forces/Tires/TireRR ==
  note: Insert your tire model here.
  Sync_In : Inport
  Load : Inport  Port=2
  vxtrans : Inport  Port=3
  vytrans : Inport  Port=4
  Rim_rotv : Inport  Port=5
  Rim_turnv : Inport  Port=6
  InclinAngle : Inport  Port=7
  muRoad : Inport  Port=8
  Ground{1..11} (11 alike) : Ground
  Terminator{,1..6,12} (8 alike) : Terminator
  Slp : Outport
  Alpha : Outport  Port=2
  TurnSlp : Outport  Port=3
  rBelt_eff : Outport  Port=4
  vBelt : Outport  Port=5
  LongFrc : Outport  Port=6
  SideFrc : Outport  Port=7
  LoadFrc : Outport  Port=8
  OverturnTrq : Outport  Port=9
  RollResist : Outport  Port=10
  AlignTrq : Outport  Port=11
  wires:
  Ground11/1 -> vBelt/1
  Ground10/1 -> rBelt_eff/1
  Ground9/1 -> TurnSlp/1
  Rim_turnv/1 -> Terminator6/1
  Sync_In/1 -> Terminator12/1
  Ground2/1 -> Alpha/1
  Ground3/1 -> LongFrc/1
  Ground4/1 -> SideFrc/1
  Ground5/1 -> OverturnTrq/1
  vxtrans/1 -> Terminator1/1
  vytrans/1 -> Terminator2/1
  Rim_rotv/1 -> Terminator3/1
  InclinAngle/1 -> Terminator4/1
  muRoad/1 -> Terminator5/1
  Load/1 -> Terminator/1
  Ground1/1 -> Slp/1
  Ground6/1 -> LoadFrc/1
  Ground7/1 -> RollResist/1
  Ground8/1 -> AlignTrq/1

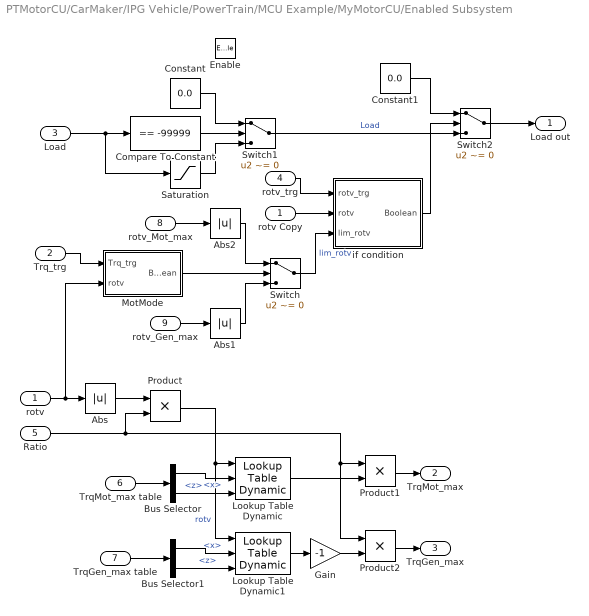
== system PTMotorCU/CarMaker/IPG Vehicle/PowerTrain/MCU Example/MyMotorCU/Enabled Subsystem ==
  rotv : Inport
  Trq_trg : Inport  Port=2
  Load : Inport  Port=3
  rotv_trg : Inport  Port=4
  Ratio : Inport  Port=5
  TrqMot_max table : Inport  Port=6
  TrqGen_max table : Inport  Port=7
  rotv_Mot_max : Inport  Port=8
  rotv_Gen_max : Inport  Port=9
  Enable : EnablePort
  Abs : Abs
  Abs1 : Abs
  Abs2 : Abs
  Bus Selector : BusSelector  OutputSignals=x,z
  Bus Selector1 : BusSelector  OutputSignals=x,z
  Compare To Constant : simulink/Logic and Bit Operations/Compare To Constant  relop===  const=-99999  OutDataTypeStr=uint8  ZeroCross=off
  Constant : Constant  Value=0.0
  Constant1 : Constant  Value=0.0
  Gain : Gain  Gain=-1
  Lookup Table Dynamic : simulink/Lookup Tables/Lookup Table Dynamic  LookUpMeth=Interpolation-Use End Values  OutDataTypeStr=float('double')  OutputDataTypeScalingMode=Specify via dialog  OutDataType=float('double')  OutScaling=2^-10  DoSatur=off
  Lookup Table Dynamic1 : simulink/Lookup Tables/Lookup Table Dynamic  LookUpMeth=Interpolation-Use End Values  OutDataTypeStr=float('double')  OutputDataTypeScalingMode=Specify via dialog  OutDataType=float('double')  OutScaling=2^-10  DoSatur=off
  MotMode : Subsystem
  Product : Product  RndMeth=Zero
  Product1 : Product  RndMeth=Zero
  Product2 : Product  RndMeth=Zero
  Saturation : Saturate  UpperLimit=1  LowerLimit=-1
  Switch : Switch  Criteria=u2 ~= 0
  Switch1 : Switch  Criteria=u2 ~= 0
  Switch2 : Switch  Criteria=u2 ~= 0
  if condition : Subsystem
  rotv Copy : InportShadow
  Load out : Outport
  TrqMot_max : Outport  Port=2
  TrqGen_max : Outport  Port=3
  wires:
  rotv Copy/1 -> if condition/2(rotv)
  Bus Selector/2 -> Lookup Table Dynamic/3  "<z>"
  Lookup Table Dynamic/1 -> Product1/2
  Abs2/1 -> Switch/1
  Abs1/1 -> Switch/3
  Product/1 -> Lookup Table Dynamic1/1, Lookup Table Dynamic/1  "rotv"
  rotv_trg/1 -> if condition/1(rotv_trg)
  if condition/1(Boolean) -> Switch2/2
  Switch1/1 -> Switch2/3  "Load"
  Constant1/1 -> Switch2/1
  Switch2/1 -> Load out/1
  Saturation/1 -> Switch1/3
  Constant/1 -> Switch1/1
  Compare To Constant/1 -> Switch1/2
  Load/1 -> Saturation/1, Compare To Constant/1
  Trq_trg/1 -> MotMode/1(Trq_trg)
  MotMode/1(Boolean) -> Switch/2
  Gain/1 -> Product2/2
  Product2/1 -> TrqGen_max/1
  Product1/1 -> TrqMot_max/1
  Switch/1 -> if condition/3(lim_rotv)  "lim_rotv"
  rotv_Mot_max/1 -> Abs2/1
  rotv_Gen_max/1 -> Abs1/1
  Lookup Table Dynamic1/1 -> Gain/1
  Bus Selector1/2 -> Lookup Table Dynamic1/3  "<z>"
  Bus Selector1/1 -> Lookup Table Dynamic1/2  "<x>"
  TrqGen_max table/1 -> Bus Selector1/1
  Bus Selector/1 -> Lookup Table Dynamic/2  "<x>"
  TrqMot_max table/1 -> Bus Selector/1
  Abs/1 -> Product/1
  Ratio/1 -> Product1/1, Product2/1, Product/2
  rotv/1 -> MotMode/2(rotv), Abs/1

== system PTMotorCU/CarMaker/IPG Vehicle/PowerTrain/MCU Example/MyMotorCU/ReturnZero ==
  Enable : EnablePort
  Bus Creator : BusCreator  Inputs=3
  Constant : Constant  Value=0.0
  Constant1 : Constant  Value=0.0
  Constant2 : Constant  Value=0.0
  Signal Conversion : SignalConversion  ConversionOutput=Bus copy  OverrideOpt=off
  ReturnZero : Outport
  wires:
  Signal Conversion/1 -> ReturnZero/1
  Constant2/1 -> Bus Creator/3  "TrqGen_max"
  Constant1/1 -> Bus Creator/2  "TrqMot_max"
  Constant/1 -> Bus Creator/1  "Load"
  Bus Creator/1 -> Signal Conversion/1

== system PTMotorCU/CarMaker/IPG Vehicle/PowerTrain/MCU Example/PTMotorCU_In/CreateBus MCU ISGIn ==
  In : Inport
  BusCreator : BusCreator  Inputs=5
  Demux : Demux  Outputs=5
  Out : Outport
  wires:
  Demux/5 -> BusCreator/5  "MCU ISGIn PwrElec"
  Demux/4 -> BusCreator/4  "MCU ISGIn rotv"
  Demux/3 -> BusCreator/3  "MCU ISGIn rotv_trg"
  Demux/2 -> BusCreator/2  "MCU ISGIn Trq"
  Demux/1 -> BusCreator/1  "MCU ISGIn Trq_trg"
  BusCreator/1 -> Out/1
  In/1 -> Demux/1

== system PTMotorCU/CarMaker/IPG Vehicle/PowerTrain/MCU Example/PTMotorCU_In/CreateBus MCU ISGOut ==
  In : Inport
  BusCreator : BusCreator  Inputs=1
  Demux : Demux  Outputs=1
  Out : Outport
  wires:
  Demux/1 -> BusCreator/1  "MCU ISGIn Load"
  BusCreator/1 -> Out/1
  In/1 -> Demux/1

== system PTMotorCU/CarMaker/IPG Vehicle/PowerTrain/MCU Example/PTMotorCU_In/CreateBus MCU Ignition ==
  In : Inport
  BusCreator : BusCreator  Inputs=1
  Demux : Demux  Outputs=1
  Out : Outport
  wires:
  Demux/1 -> BusCreator/1  "MCU Ignition"
  BusCreator/1 -> Out/1
  In/1 -> Demux/1

== system PTMotorCU/CarMaker/IPG Vehicle/PowerTrain/MCU Example/PTMotorCU_In/CreateBus MCU MotorIn0 ==
  In : Inport
  BusCreator : BusCreator  Inputs=5
  Demux : Demux  Outputs=5
  Out : Outport
  wires:
  Demux/5 -> BusCreator/5  "MCU MotorIn0 PwrElec"
  Demux/4 -> BusCreator/4  "MCU MotorIn0 rotv"
  Demux/3 -> BusCreator/3  "MCU MotorIn0 rotv_trg"
  Demux/2 -> BusCreator/2  "MCU MotorIn0 Trq"
  Demux/1 -> BusCreator/1  "MCU MotorIn0 Trq_trg"
  BusCreator/1 -> Out/1
  In/1 -> Demux/1

== system PTMotorCU/CarMaker/IPG Vehicle/PowerTrain/MCU Example/PTMotorCU_In/CreateBus MCU MotorIn1 ==
  In : Inport
  BusCreator : BusCreator  Inputs=5
  Demux : Demux  Outputs=5
  Out : Outport
  wires:
  Demux/5 -> BusCreator/5  "MCU MotorIn1 PwrElec"
  Demux/4 -> BusCreator/4  "MCU MotorIn1 rotv"
  Demux/3 -> BusCreator/3  "MCU MotorIn1 rotv_trg"
  Demux/2 -> BusCreator/2  "MCU MotorIn1 Trq"
  Demux/1 -> BusCreator/1  "MCU MotorIn1 Trq_trg"
  BusCreator/1 -> Out/1
  In/1 -> Demux/1

== system PTMotorCU/CarMaker/IPG Vehicle/PowerTrain/MCU Example/PTMotorCU_In/CreateBus MCU MotorIn2 ==
  In : Inport
  BusCreator : BusCreator  Inputs=5
  Demux : Demux  Outputs=5
  Out : Outport
  wires:
  Demux/5 -> BusCreator/5  "MCU MotorIn2 PwrElec"
  Demux/4 -> BusCreator/4  "MCU MotorIn2 rotv"
  Demux/3 -> BusCreator/3  "MCU MotorIn2 rotv_trg"
  Demux/2 -> BusCreator/2  "MCU MotorIn2 Trq"
  Demux/1 -> BusCreator/1  "MCU MotorIn2 Trq_trg"
  BusCreator/1 -> Out/1
  In/1 -> Demux/1

== system PTMotorCU/CarMaker/IPG Vehicle/PowerTrain/MCU Example/PTMotorCU_In/CreateBus MCU MotorIn3 ==
  In : Inport
  BusCreator : BusCreator  Inputs=5
  Demux : Demux  Outputs=5
  Out : Outport
  wires:
  Demux/5 -> BusCreator/5  "MCU MotorIn3 PwrElec"
  Demux/4 -> BusCreator/4  "MCU MotorIn3 rotv"
  Demux/3 -> BusCreator/3  "MCU MotorIn3 rotv_trg"
  Demux/2 -> BusCreator/2  "MCU MotorIn3 Trq"
  Demux/1 -> BusCreator/1  "MCU MotorIn3 Trq_trg"
  BusCreator/1 -> Out/1
  In/1 -> Demux/1

== system PTMotorCU/CarMaker/IPG Vehicle/PowerTrain/MCU Example/PTMotorCU_In/CreateBus MCU MotorOut0 ==
  In : Inport
  BusCreator : BusCreator  Inputs=1
  Demux : Demux  Outputs=1
  Out : Outport
  wires:
  Demux/1 -> BusCreator/1  "MCU MotorOut0 Load"
  BusCreator/1 -> Out/1
  In/1 -> Demux/1

== system PTMotorCU/CarMaker/IPG Vehicle/PowerTrain/MCU Example/PTMotorCU_In/CreateBus MCU MotorOut1 ==
  In : Inport
  BusCreator : BusCreator  Inputs=1
  Demux : Demux  Outputs=1
  Out : Outport
  wires:
  Demux/1 -> BusCreator/1  "MCU MotorOut1 Load"
  BusCreator/1 -> Out/1
  In/1 -> Demux/1

== system PTMotorCU/CarMaker/IPG Vehicle/PowerTrain/MCU Example/PTMotorCU_In/CreateBus MCU MotorOut2 ==
  In : Inport
  BusCreator : BusCreator  Inputs=1
  Demux : Demux  Outputs=1
  Out : Outport
  wires:
  Demux/1 -> BusCreator/1  "MCU MotorOut2 Load"
  BusCreator/1 -> Out/1
  In/1 -> Demux/1

== system PTMotorCU/CarMaker/IPG Vehicle/PowerTrain/MCU Example/PTMotorCU_In/CreateBus MCU MotorOut3 ==
  In : Inport
  BusCreator : BusCreator  Inputs=1
  Demux : Demux  Outputs=1
  Out : Outport
  wires:
  Demux/1 -> BusCreator/1  "MCU MotorOut3 Load"
  BusCreator/1 -> Out/1
  In/1 -> Demux/1

== system PTMotorCU/CarMaker/IPG Vehicle/PowerTrain/MCU Example/PTMotorCU_In/CreateBus MCU_Cfg ISG ==
  In : Inport
  BusCreator : BusCreator  Inputs=3
  Demux : Demux  Outputs=3
  Out : Outport
  wires:
  Demux/3 -> BusCreator/3  "MCU_Cfg ISG rotv_Gen_max"
  Demux/2 -> BusCreator/2  "MCU_Cfg ISG rotv_Mot_max"
  Demux/1 -> BusCreator/1  "MCU_Cfg ISG Ratio"
  BusCreator/1 -> Out/1
  In/1 -> Demux/1

== system PTMotorCU/CarMaker/IPG Vehicle/PowerTrain/MCU Example/PTMotorCU_In/CreateBus MCU_Cfg Misc ==
  In : Inport
  BusCreator : BusCreator  Inputs=1
  Demux : Demux  Outputs=1
  Out : Outport
  wires:
  Demux/1 -> BusCreator/1  "MCU_Cfg nMotor"
  BusCreator/1 -> Out/1
  In/1 -> Demux/1

== system PTMotorCU/CarMaker/IPG Vehicle/PowerTrain/MCU Example/PTMotorCU_In/CreateBus MCU_Cfg Motor0 ==
  In : Inport
  BusCreator : BusCreator  Inputs=3
  Demux : Demux  Outputs=3
  Out : Outport
  wires:
  Demux/3 -> BusCreator/3  "MCU_Cfg Motor0 rotv_Gen_max"
  Demux/2 -> BusCreator/2  "MCU_Cfg Motor0 rotv_Mot_max"
  Demux/1 -> BusCreator/1  "MCU_Cfg Motor0 Ratio"
  BusCreator/1 -> Out/1
  In/1 -> Demux/1

== system PTMotorCU/CarMaker/IPG Vehicle/PowerTrain/MCU Example/PTMotorCU_In/CreateBus MCU_Cfg Motor1 ==
  In : Inport
  BusCreator : BusCreator  Inputs=3
  Demux : Demux  Outputs=3
  Out : Outport
  wires:
  Demux/3 -> BusCreator/3  "MCU_Cfg Motor1 rotv_Gen_max"
  Demux/2 -> BusCreator/2  "MCU_Cfg Motor1 rotv_Mot_max"
  Demux/1 -> BusCreator/1  "MCU_Cfg Motor1 Ratio"
  BusCreator/1 -> Out/1
  In/1 -> Demux/1

== system PTMotorCU/CarMaker/IPG Vehicle/PowerTrain/MCU Example/PTMotorCU_In/CreateBus MCU_Cfg Motor2 ==
  In : Inport
  BusCreator : BusCreator  Inputs=3
  Demux : Demux  Outputs=3
  Out : Outport
  wires:
  Demux/3 -> BusCreator/3  "MCU_Cfg Motor2 rotv_Gen_max"
  Demux/2 -> BusCreator/2  "MCU_Cfg Motor2 rotv_Mot_max"
  Demux/1 -> BusCreator/1  "MCU_Cfg Motor2 Ratio"
  BusCreator/1 -> Out/1
  In/1 -> Demux/1

== system PTMotorCU/CarMaker/IPG Vehicle/PowerTrain/MCU Example/PTMotorCU_In/CreateBus MCU_Cfg Motor3 ==
  In : Inport
  BusCreator : BusCreator  Inputs=3
  Demux : Demux  Outputs=3
  Out : Outport
  wires:
  Demux/3 -> BusCreator/3  "MCU_Cfg Motor3 rotv_Gen_max"
  Demux/2 -> BusCreator/2  "MCU_Cfg Motor3 rotv_Mot_max"
  Demux/1 -> BusCreator/1  "MCU_Cfg Motor3 Ratio"
  BusCreator/1 -> Out/1
  In/1 -> Demux/1

== system PTMotorCU/CarMaker/IPG Vehicle/PowerTrain/MCU Example/MyMotorCU/Enabled Subsystem/MotMode ==
  Trq_trg : Inport
  rotv : Inport  Port=2
  Compare To Zero : simulink/Logic and Bit Operations/Compare To Zero  relop=<  OutDataTypeStr=uint8  ZeroCross=off
  Compare To Zero1 : simulink/Logic and Bit Operations/Compare To Zero  relop=>=  OutDataTypeStr=uint8  ZeroCross=off
  Gain : Gain  Gain=-1
  Logical Operator : Logic  AllPortsSameDT=off  OutDataTypeStr=boolean
  Logical Operator1 : Logic  AllPortsSameDT=off  OutDataTypeStr=boolean
  Logical Operator2 : Logic  Operator=OR  AllPortsSameDT=off  OutDataTypeStr=boolean
  Relational Operator2 : RelationalOperator  OutDataTypeStr=boolean
  Relational Operator3 : RelationalOperator  Operator=<  OutDataTypeStr=boolean
  limrotv : Constant  Value=0.5
  Boolean : Outport
  wires:
  Gain/1 -> Relational Operator2/2
  Relational Operator3/1 -> Logical Operator1/2
  limrotv/1 -> Gain/1, Relational Operator3/2
  rotv/1 -> Relational Operator3/1, Relational Operator2/1
  Relational Operator2/1 -> Logical Operator/2
  Compare To Zero/1 -> Logical Operator1/1
  Trq_trg/1 -> Compare To Zero/1, Compare To Zero1/1
  Compare To Zero1/1 -> Logical Operator/1
  Logical Operator1/1 -> Logical Operator2/2
  Logical Operator/1 -> Logical Operator2/1
  Logical Operator2/1 -> Boolean/1

== system PTMotorCU/CarMaker/IPG Vehicle/PowerTrain/MCU Example/MyMotorCU/Enabled Subsystem/if condition ==
  rotv_trg : Inport
  rotv : Inport  Port=2
  lim_rotv : Inport  Port=3
  Abs : Abs
  Compare To Constant : simulink/Logic and Bit Operations/Compare To Constant  relop===  const=-99999  OutDataTypeStr=boolean  ZeroCross=off
  Logical Operator : Logic  AllPortsSameDT=off  OutDataTypeStr=boolean
  Relational Operator : RelationalOperator  Operator=>  OutDataTypeStr=boolean
  Boolean : Outport
  wires:
  Abs/1 -> Relational Operator/1
  rotv/1 -> Abs/1
  lim_rotv/1 -> Relational Operator/2
  Relational Operator/1 -> Logical Operator/1
  Compare To Constant/1 -> Logical Operator/2
  rotv_trg/1 -> Compare To Constant/1
  Logical Operator/1 -> Boolean/1
